simulink library "rtwdemo_configurable_source"  (Simulink 7.6)
settings: Solver=ode45  SolverMode=SingleTasking  StartTime=0.0  StopTime=10.0  RelTol=1e-3
libraries: rtwdemo_configurable_source x1
settings Model: Creator=The MathWorks Inc.  ExtModeAutoUpdateStatusClock=off

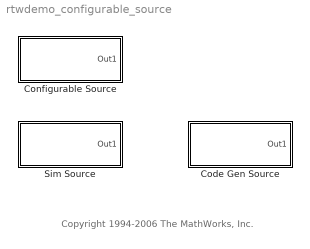
== system rtwdemo_configurable_source ==
  note: Copyright 1994-2006 The MathWorks, Inc.
  Code Gen Source : Subsystem
  Configurable Source : Subsystem  BlockChoice=Sim Source
      mask init:
      | if rtwenvironmentmode(bdroot(gcbh))
      | 	set_param(gcbh, 'BlockChoice', 'Sim Source');
      | else
      | 	set_param(gcbh, 'BlockChoice', 'Code Gen Source');
      | end
      settings: TemplateBlock=self  MemberBlocks=Code Gen Source,Sim Source
      mask Display: disp('Configurable Source');
  Sim Source : Subsystem

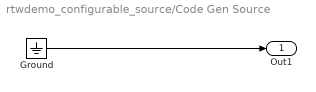
== system rtwdemo_configurable_source/Code Gen Source ==
  Ground : Ground
  Out1 : Outport
  wires:
  Ground/1 -> Out1/1

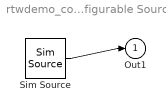
== system rtwdemo_configurable_source/Configurable Source ==
  Sim Source : rtwdemo_configurable_source/Sim Source  SystemSampleTime=-1
  Out1 : Outport
  wires:
  Sim Source/1 -> Out1/1

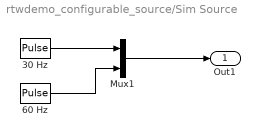
== system rtwdemo_configurable_source/Sim Source ==
  30 Hz : DiscretePulseGenerator  SampleTime=1/30  VectorParams1D=off
  60 Hz : DiscretePulseGenerator  Period=4  PulseWidth=2  SampleTime=1/60
  Mux1 : Mux  Inputs=2
  Out1 : Outport
  wires:
  60 Hz/1 -> Mux1/2
  30 Hz/1 -> Mux1/1
  Mux1/1 -> Out1/1
